simulink model "prelab1a"  (Simulink 7.8)
settings: Solver=ode45  StartTime=0.0  StopTime=10.0  RelTol=1e-3
libraries: simulink x4
settings Model: Creator=Embed_Sys_course  LastModifiedBy=Embed_Sys_course

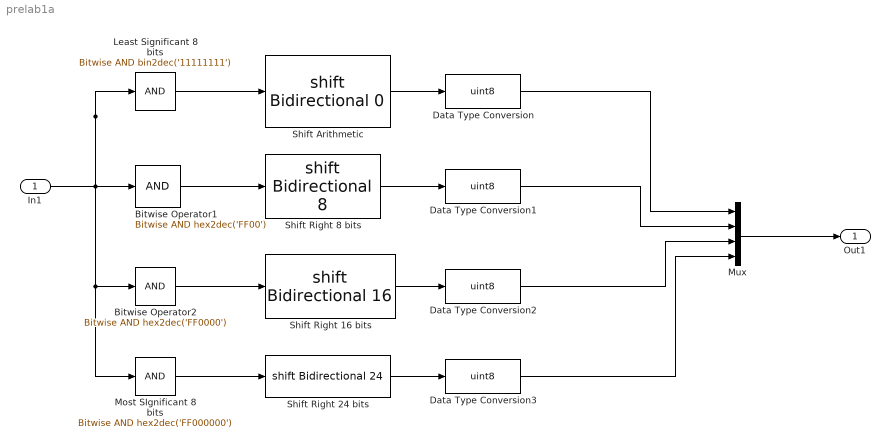
== system prelab1a ==
  In1 : Inport
  Bitwise Operator1 : simulink/Logic and Bit Operations/Bitwise Operator  logicop=AND  UseBitMask=on  BitMask=hex2dec('FF00')  BitMaskRealWorld=Stored Integer
  Bitwise Operator2 : simulink/Logic and Bit Operations/Bitwise Operator  logicop=AND  UseBitMask=on  BitMask=hex2dec('FF0000')  BitMaskRealWorld=Stored Integer
  Data Type Conversion{,1..3} (4 alike) : DataTypeConversion  OutDataTypeStr=uint8
  Least Significant 8 bits : simulink/Logic and Bit Operations/Bitwise Operator  logicop=AND  UseBitMask=on  BitMask=bin2dec('11111111')  BitMaskRealWorld=Stored Integer
  Most SIgnificant 8 bits : simulink/Logic and Bit Operations/Bitwise Operator  logicop=AND  UseBitMask=on  BitMask=hex2dec('FF000000')  BitMaskRealWorld=Stored Integer
  Mux : Mux
  Shift Arithmetic : ArithShift
  Shift Right 16 bits : ArithShift  BitShiftNumber=16
  Shift Right 24 bits : ArithShift  BitShiftNumber=24
  Shift Right 8 bits : ArithShift  BitShiftNumber=8
  Out1 : Outport
  wires:
  Least Significant 8 bits/1 -> Shift Arithmetic/1
  In1/1 -> Least Significant 8 bits/1, Bitwise Operator1/1, Bitwise Operator2/1, Most SIgnificant 8 bits/1
  Bitwise Operator1/1 -> Shift Right 8 bits/1
  Bitwise Operator2/1 -> Shift Right 16 bits/1
  Most SIgnificant 8 bits/1 -> Shift Right 24 bits/1
  Shift Arithmetic/1 -> Data Type Conversion/1
  Shift Right 8 bits/1 -> Data Type Conversion1/1
  Shift Right 16 bits/1 -> Data Type Conversion2/1
  Shift Right 24 bits/1 -> Data Type Conversion3/1
  Data Type Conversion/1 -> Mux/1
  Data Type Conversion1/1 -> Mux/2
  Data Type Conversion2/1 -> Mux/3
  Data Type Conversion3/1 -> Mux/4
  Mux/1 -> Out1/1
